simulink model "Obtencion_Datos"  (R2021a)
settings: Solver=VariableStepAuto  StartTime=0.0  StopTime=inf  RelTol=1e-3
undefined symbols (not defined in the file or in its folder): Ir, T
libraries: spsDiodeLib x5, spsPVArrayLib x5, simulink x2, spsControlledVoltageSourceLib x1, spsCurrentMeasurementLib x1, spsVoltageMeasurementLib x1, spspowerguiLib x1
settings Model: Creator=nacho  LastModifiedBy=nacho

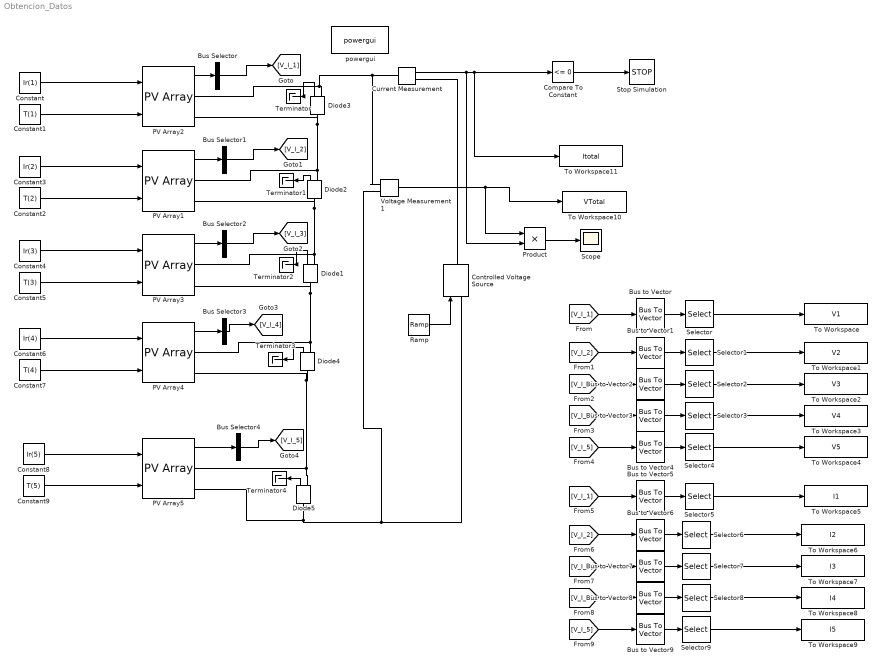
== system Obtencion_Datos ==
  Bus Selector{,1..4} (5 alike) : BusSelector  OutputSignals=V_PV,I_PV  OutputAsBus=on
  Bus to Vector{,1..9} (10 alike) : BusToVector
  Compare To Constant : simulink/Logic and Bit Operations/Compare To Constant  relop=<=  const=0  OutDataTypeStr=boolean
  Constant : Constant  Value=Ir(1)
  Constant1 : Constant  Value=T(1)
  Constant2 : Constant  Value=T(2)
  Constant3 : Constant  Value=Ir(2)
  Constant4 : Constant  Value=Ir(3)
  Constant5 : Constant  Value=T(3)
  Constant6 : Constant  Value=Ir(4)
  Constant7 : Constant  Value=T(4)
  Constant8 : Constant  Value=Ir(5)
  Constant9 : Constant  Value=T(5)
  Controlled Voltage Source : spsControlledVoltageSourceLib/Controlled Voltage Source  Initialize=on  Source_Type=DC  Amplitude=0  Phase=0  Frequency=0  Measurements=Voltage
  Current Measurement : spsCurrentMeasurementLib/Current Measurement  PhasorSimulation=off  OutputType=Complex  PSBequivalent=0
  Diode{1..5} (5 alike) : spsDiodeLib/Diode  Ron=0.001  Lon=0  Vf=0.8  IC=0  UseSnubber=0  Rs=500  Cs=250e-9  Measurements=on
  PV Array{1..5} (5 alike) : spsPVArrayLib/PV Array  Npar=1  Nser=1  PlotType=one module @ 25 deg.C & specified irradiances  S_vec="[ 1000  500  100 ]"  Temp_C_vec="[ 45 25  ]"  ModuleName=Apollo Solar Energy ASEC-325G6S  PlotWhenSelected=off  Pm=324.9897  Ncell=72  Voc=45.48  Isc=9.39  Vm=35.99  Im=9.03  beta_Voc_pc=-0.343  alpha_Isc_pc=0.072897  beta_Voc=-0.156  alpha_Isc=0.006845  IL=9.5248  I0=1.7974e-10  nI=0.99584  Rsh=992.2435  Rs=0.45891  RobustModel=off  RobustCellTemperature=313.3991  BAL=on  Tc=1e-6  Tfilter=5e-5
  Product : Product
  Ramp : simulink/Sources/Ramp  slope=500  start=0  InitialOutput=0
  Scope : Scope
  Selector{,1..4} (5 alike) : Selector  InputPortWidth=2  IndexOptions=Index vector (dialog)  Indices=[1]  OutputSizes=1
  Selector{5..9} (5 alike) : Selector  InputPortWidth=2  IndexOptions=Index vector (dialog)  Indices=[2]  OutputSizes=1
  Stop Simulation : Stop
  Terminator{,1..4} (5 alike) : Terminator
  To Workspace : ToWorkspace  VariableName=V1  SampleTime=-1
  To Workspace1 : ToWorkspace  VariableName=V2  SampleTime=-1
  To Workspace10 : ToWorkspace  VariableName=VTotal  SampleTime=-1
  To Workspace11 : ToWorkspace  VariableName=Itotal  SampleTime=-1
  To Workspace2 : ToWorkspace  VariableName=V3  SampleTime=-1
  To Workspace3 : ToWorkspace  VariableName=V4  SampleTime=-1
  To Workspace4 : ToWorkspace  VariableName=V5  SampleTime=-1
  To Workspace5 : ToWorkspace  VariableName=I1  SampleTime=-1
  To Workspace6 : ToWorkspace  VariableName=I2  SampleTime=-1
  To Workspace7 : ToWorkspace  VariableName=I3  SampleTime=-1
  To Workspace8 : ToWorkspace  VariableName=I4  SampleTime=-1
  To Workspace9 : ToWorkspace  VariableName=I5  SampleTime=-1
  Voltage Measurement1 : spsVoltageMeasurementLib/Voltage Measurement  PhasorSimulation=off  OutputType=Complex  PSBequivalent=0
  powergui : spspowerguiLib/powergui  Priority=1  SimulationMode=Continuous  SampleTime=50e-6  frequency=60  Iterations=50  frequencyindice=0  Pbase=100e6  ErrMax=1e-4  UnitsV=kV  UnitsW=MW  buscounter=0  FunctionMessages=off  echomessages=off  EnableUseOfTLC=off  CurrentSourceSwitches=off  DisableSnubberDevices=off  DisableRonSwitches=off  DisableVfSwitches=off  DisplayEquations=off  AutomaticDiscreteSolvers=off  SolverType=Tustin/Backward Euler (TBE)  Interpol=off  ExternalGateDelay=off  methode=off  Ts=100  x0status=blocks  SPID=on  SwTol=0  HookPort=off  NonlinearTolerance=1e-4  nMaxIteration=100  ContinueOnMaxIteration=off  RestoreLinks=warning  ResistiveCurrentMeasurement=off  Frange=[0:2:500]  Ylog=off  Xlog=on  ShowGrid=off  save=off  variable=ZData  structure=0  ZoomFFT=off  StartTime=0.0  cycles=1  DisplayStyle=1  fundamental=60  FreqAxis=off  MaxFrequency=1000  frequencyindicesteady=1  RmsSteady=1  display=off
  wires:
  Ramp/1 -> Controlled Voltage Source/1
  Compare To Constant/1 -> Stop Simulation/1
  Current Measurement/1 -> Product/2, To Workspace11/1, Compare To Constant/1
  Constant/1 -> PV Array2/1
  Constant1/1 -> PV Array2/2
  Constant2/1 -> PV Array1/2
  Constant3/1 -> PV Array1/1
  Constant4/1 -> PV Array3/1
  Constant5/1 -> PV Array3/2
  Constant6/1 -> PV Array4/1
  Constant7/1 -> PV Array4/2
  Constant8/1 -> PV Array5/1
  Constant9/1 -> PV Array5/2
  PV Array1/1 -> Bus Selector1/1
  PV Array3/1 -> Bus Selector2/1
  PV Array4/1 -> Bus Selector3/1
  PV Array2/1 -> Bus Selector/1
  Bus Selector/1 -> [V_I_1]
  Bus Selector1/1 -> [V_I_2]
  Bus Selector2/1 -> [V_I_3]
  Bus Selector3/1 -> [V_I_4]
  Bus Selector4/1 -> [V_I_5]
  PV Array5/1 -> Bus Selector4/1
  [V_I_1] -> Bus to Vector/1
  [V_I_2] -> Bus to Vector1/1
  [V_I_3] -> Bus to Vector2/1
  [V_I_4] -> Bus to Vector3/1
  [V_I_5] -> Bus to Vector4/1
  Bus to Vector/1 -> Selector/1
  Bus to Vector1/1 -> Selector1/1
  Bus to Vector2/1 -> Selector2/1
  Bus to Vector3/1 -> Selector3/1
  Bus to Vector4/1 -> Selector4/1
  Bus to Vector6/1 -> Selector6/1
  Bus to Vector5/1 -> Selector5/1
  Bus to Vector9/1 -> Selector9/1
  [V_I_2] -> Bus to Vector6/1
  Bus to Vector7/1 -> Selector7/1
  [V_I_1] -> Bus to Vector5/1
  Bus to Vector8/1 -> Selector8/1
  [V_I_4] -> Bus to Vector8/1
  [V_I_5] -> Bus to Vector9/1
  [V_I_3] -> Bus to Vector7/1
  Selector/1 -> To Workspace/1
  Selector1/1 -> To Workspace1/1
  Selector2/1 -> To Workspace2/1
  Selector3/1 -> To Workspace3/1
  Selector4/1 -> To Workspace4/1
  Selector8/1 -> To Workspace8/1
  Selector5/1 -> To Workspace5/1
  Selector7/1 -> To Workspace7/1
  Selector9/1 -> To Workspace9/1
  Selector6/1 -> To Workspace6/1
  Voltage Measurement1/1 -> Product/1, To Workspace10/1
  Product/1 -> Scope/1
  Diode3/1 -> Terminator/1
  Diode2/1 -> Terminator1/1
  Diode1/1 -> Terminator2/1
  Diode4/1 -> Terminator3/1
  Diode5/1 -> Terminator4/1
  connections:
  PV Array1/RConn2 -- Diode1/RConn1 -- PV Array3/RConn1 -- Diode2/LConn1
  PV Array2/RConn2 -- Diode3/LConn1 -- Diode2/RConn1 -- PV Array1/RConn1
  Diode3/RConn1 -- Voltage Measurement1/LConn1 -- Current Measurement/LConn1 -- PV Array2/RConn1
  PV Array5/RConn1 -- Diode5/RConn1 -- Diode4/LConn1 -- PV Array4/RConn2
  PV Array3/RConn2 -- Diode4/RConn1 -- PV Array4/RConn1 -- Diode1/LConn1
  PV Array5/RConn2 -- Voltage Measurement1/LConn2 -- Controlled Voltage Source/LConn1 -- Diode5/LConn1
  Current Measurement/RConn1 -- Controlled Voltage Source/RConn1
